simulink model "AC_model"  (R2022a)
settings: Solver=VariableStepAuto  StartTime=0.0  StopTime=300  RelTol=1e-3
undefined symbols (not defined in the file or in its folder): DiscIntNeverNeededParam
libraries: rllib x1, commrandsrc3 x1
settings Model: Creator=OPCUSER  LastModifiedBy=bowen
settings SolverCC: AlgebraicLoopSolver=TrustRegion
settings DebuggingCC: UnconnectedInputMsg=warning  UnconnectedOutputMsg=warning  UnconnectedLineMsg=warning  SFMachineParentedDataDiag=warning
settings SFSimCC: CustomCodeUndefinedFunction=UseInterfaceOnly

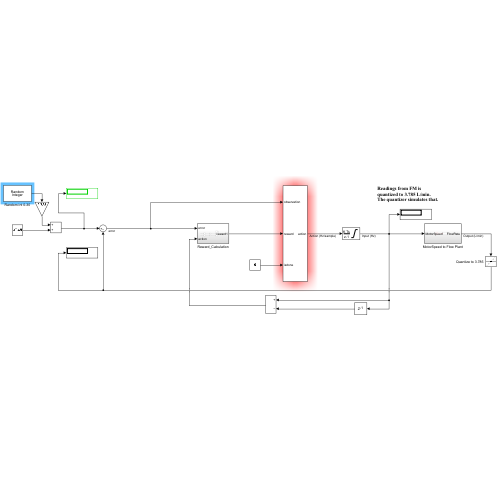
[thumbnail: Simulink's stored preview of the top-level diagram]
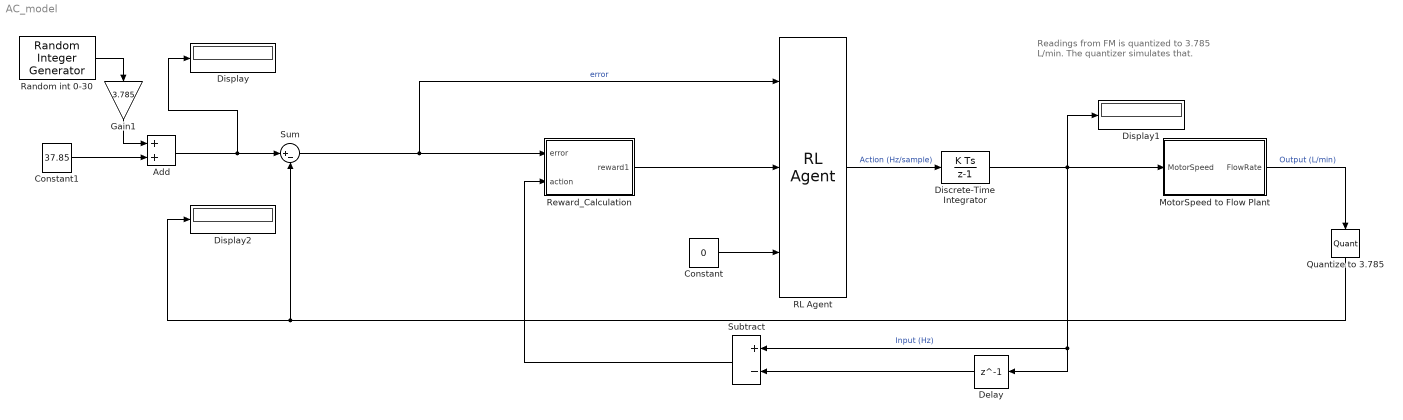
== system AC_model ==
  note: Readings from FM is quantized to 3.785 L/min.
      | The quantizer simulates that.
  Add : Sum
  Constant : Constant  Value=0
  Constant1 : Constant  Value=37.85
  Delay : Delay  DelayLength=1  InitialCondition=0
  Discrete-Time Integrator : DiscreteIntegrator  gainval=1  InitialCondition=10  SampleTime=-1  LimitOutput=on  UpperSaturationLimit=55  LowerSaturationLimit=10  ICPrevOutput=DiscIntNeverNeededParam  ICPrevScaledInput=DiscIntNeverNeededParam
  Display : Display
  Display1 : Display
  Display2 : Display
  Gain1 : Gain  Gain=3.785
  MotorSpeed to Flow Plant : Subsystem
  Quantize to 3.785 : Quantizer  QuantizationInterval=3.785
  RL Agent : rllib/RL Agent  Agent=agent  ExternalActionAsInput=off  ProvideLastAction=off  ProvideCumRwd=off  TreatAsDirectFeedthrough=on  UseStrictObservationDataTypes=off
  Random int 0-30 : commrandsrc3/Random Integer Generator  SetSize=30  SeedSource=Auto  Seed=0  SampleTime=45  SamplesPerFrame=1  OutputDataType=double  SimulateUsing=Interpreted execution
  Reward_Calculation : Subsystem
  Subtract : Sum  Inputs=+-
  Sum : Sum  Inputs=|+-
  wires:
  Quantize to 3.785/1 -> Display2/1, Sum/2
  Discrete-Time Integrator/1 -> Delay/1, Subtract/1, Display1/1, MotorSpeed to Flow Plant/1(MotorSpeed)  "Input (Hz)"
  MotorSpeed to Flow Plant/1(FlowRate) -> Quantize to 3.785/1  "Output (L/min)"
  Sum/1 -> RL Agent/1, Reward_Calculation/1(error)  "error"
  RL Agent/1 -> Discrete-Time Integrator/1  "Action (Hz/sample)"
  Constant/1 -> RL Agent/3
  Reward_Calculation/1(reward1) -> RL Agent/2
  Delay/1 -> Subtract/2
  Subtract/1 -> Reward_Calculation/2(action)
  Gain1/1 -> Add/1
  Random int 0-30/1 -> Gain1/1
  Constant1/1 -> Add/2
  Add/1 -> Sum/1, Display/1

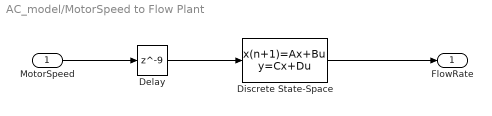
== system AC_model/MotorSpeed to Flow Plant ==
  MotorSpeed : Inport
  Delay : Delay  DelayLength=9  InitialCondition=0  SampleTime=0.15
  Discrete State-Space : DiscreteStateSpace  A=0.882  B=0.36  D=0  SampleTime=0.15
  FlowRate : Outport  VectorParamsAs1DForOutWhenUnconnected=off
  wires:
  Delay/1 -> Discrete State-Space/1
  MotorSpeed/1 -> Delay/1
  Discrete State-Space/1 -> FlowRate/1

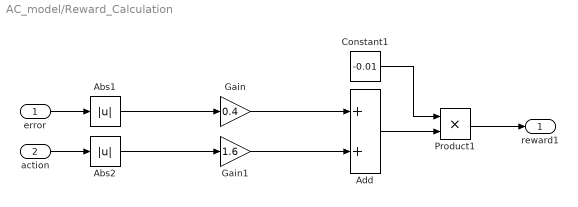
== system AC_model/Reward_Calculation ==
  error : Inport
  action : Inport  Port=2
  Abs1 : Abs  SaturateOnIntegerOverflow=off
  Abs2 : Abs  SaturateOnIntegerOverflow=off
  Add : Sum
  Constant1 : Constant  Value=-0.01
  Gain : Gain  Gain=0.4
  Gain1 : Gain  Gain=1.6
  Product1 : Product
  reward1 : Outport  VectorParamsAs1DForOutWhenUnconnected=off
  wires:
  Product1/1 -> reward1/1
  error/1 -> Abs1/1
  Abs1/1 -> Gain/1
  Constant1/1 -> Product1/1
  action/1 -> Abs2/1
  Abs2/1 -> Gain1/1
  Add/1 -> Product1/2
  Gain1/1 -> Add/2
  Gain/1 -> Add/1
